simulink model "LIN_Edge"  (R2016b)
settings: Solver=FixedStepAuto  StartTime=0.0  StopTime=10  FixedStep=0.001  RelTol=1e-3
values from neighbouring files (symbols this model uses):
  A = [0, 1, 0; m*l_C*g*sqrt(2)/I_K, -C_psi/I_K, C_psi/I_K; 0, C_psi/I_R, -C_psi/I_R]    [ParameterInit.m]
  Ad = SSd.A    [ParameterInit.m]
  B = [0; -1/I_K; 1/I_R]    [ParameterInit.m]
  Bd = SSd.B    [ParameterInit.m]
  C = [0, 1, 0; 0, 0, 1]    [ParameterInit.m]
  Cd = SSd.C    [ParameterInit.m]
  Ta = 0.02    [ParameterInit.m]
undefined symbols (not defined in the file or in its folder): Kd, Ld, x_0, x_offset
libraries: simulink x1
settings Model: Creator=michael  LastModifiedBy=ich

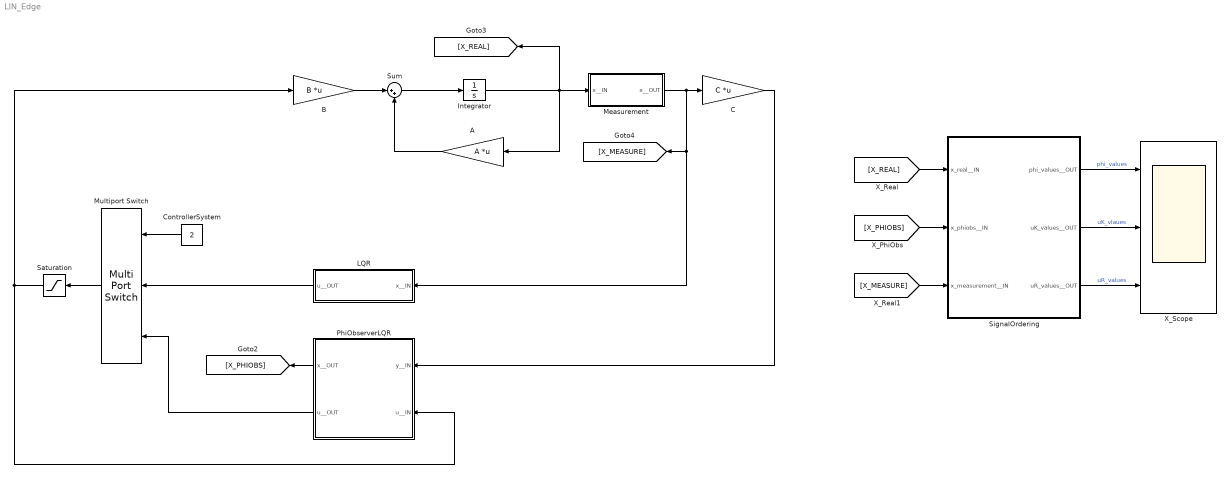
== system LIN_Edge ==
  A : Gain  Gain=A  Multiplication=Matrix(K*u) (u vector)
  B : Gain  Gain=B  Multiplication=Matrix(K*u) (u vector)
  C : Gain  Gain=C  Multiplication=Matrix(K*u) (u vector)
  ControllerSystem : Constant  Value=2
  Integrator : Integrator  InitialCondition=x_0
  LQR : Subsystem
  Measurement : Subsystem
  Multiport Switch : MultiPortSwitch  Inputs=2
  PhiObserverLQR : Subsystem
  Saturation : Saturate  UpperLimit=0.11  LowerLimit=-0.11
  SignalOrdering : Subsystem
  Sum : Sum  Inputs=|++
  X_Scope : Scope  NumInputPorts=3
  wires:
  B/1 -> Sum/1
  Sum/1 -> Integrator/1
  A/1 -> Sum/2
  Integrator/1 -> [X_REAL], Measurement/1(x__IN), A/1
  Measurement/1(x__OUT) -> C/1, LQR/1(x__IN), [X_MEASURE]
  Multiport Switch/1 -> Saturation/1
  LQR/1(u__OUT) -> Multiport Switch/2
  ControllerSystem/1 -> Multiport Switch/1
  Saturation/1 -> PhiObserverLQR/2(u__IN), B/1
  PhiObserverLQR/1(x__OUT) -> [X_PHIOBS]
  C/1 -> PhiObserverLQR/1(y__IN)
  [X_REAL] -> SignalOrdering/1(x_real__IN)
  [X_PHIOBS] -> SignalOrdering/2(x_phiobs__IN)
  [X_MEASURE] -> SignalOrdering/3(x_measurement__IN)
  SignalOrdering/1(phi_values__OUT) -> X_Scope/1  "phi_values"
  SignalOrdering/2(uK_values__OUT) -> X_Scope/2  "uK_vlaues"
  SignalOrdering/3(uR_values__OUT) -> X_Scope/3  "uR_values"
  PhiObserverLQR/2(u__OUT) -> Multiport Switch/3

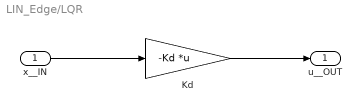
== system LIN_Edge/LQR ==
  x__IN : Inport  SampleTime=Ta
  Kd : Gain  Gain=-Kd  Multiplication=Matrix(K*u) (u vector)
  u__OUT : Outport
  wires:
  x__IN/1 -> Kd/1
  Kd/1 -> u__OUT/1

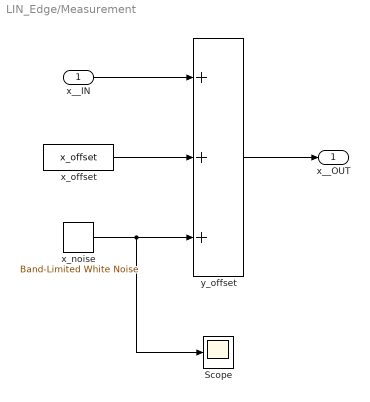
== system LIN_Edge/Measurement ==
  x__IN : Inport  SampleTime=Ta
  Scope : Scope
  x_noise : simulink/Sources/Band-Limited White Noise  Cov=y_noise  Ts=0.02  seed=[23341]
  x_offset : Constant  Value=x_offset
  y_offset : Sum  Inputs=+++
  x__OUT : Outport
  wires:
  x__IN/1 -> y_offset/1
  y_offset/1 -> x__OUT/1
  x_offset/1 -> y_offset/2
  x_noise/1 -> Scope/1, y_offset/3

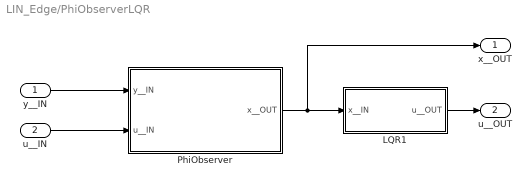
== system LIN_Edge/PhiObserverLQR ==
  y__IN : Inport
  u__IN : Inport  Port=2
  LQR1 : Subsystem
  PhiObserver : Subsystem
  x__OUT : Outport
  u__OUT : Outport  Port=2
  wires:
  LQR1/1(u__OUT) -> u__OUT/1
  PhiObserver/1(x__OUT) -> x__OUT/1, LQR1/1(x__IN)
  u__IN/1 -> PhiObserver/2(u__IN)
  y__IN/1 -> PhiObserver/1(y__IN)

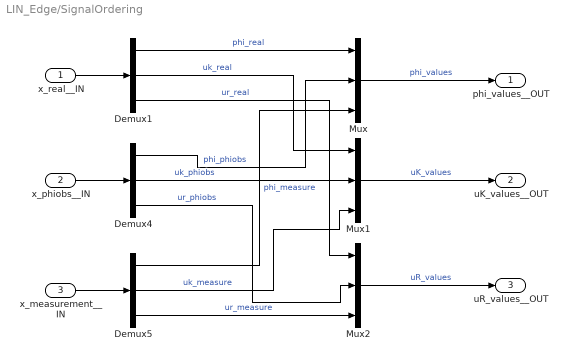
== system LIN_Edge/SignalOrdering ==
  x_real__IN : Inport
  x_phiobs__IN : Inport  Port=2
  x_measurement__IN : Inport  Port=3
  Demux1 : Demux  Outputs=3
  Demux4 : Demux  Outputs=3
  Demux5 : Demux  Outputs=3
  Mux : Mux  Inputs=3
  Mux1 : Mux  Inputs=3
  Mux2 : Mux  Inputs=3
  phi_values__OUT : Outport
  uK_values__OUT : Outport  Port=2
  uR_values__OUT : Outport  Port=3
  wires:
  Demux1/2 -> Mux1/1  "uk_real"
  Demux4/2 -> Mux1/2  "uk_phiobs"
  Demux4/3 -> Mux2/2  "ur_phiobs"
  x_real__IN/1 -> Demux1/1
  Mux/1 -> phi_values__OUT/1  "phi_values"
  Mux1/1 -> uK_values__OUT/1  "uK_values"
  Mux2/1 -> uR_values__OUT/1  "uR_values"
  Demux5/2 -> Mux1/3  "uk_measure"
  Demux1/1 -> Mux/1  "phi_real"
  x_measurement__IN/1 -> Demux5/1
  Demux4/1 -> Mux/2  "phi_phiobs"
  Demux1/3 -> Mux2/1  "ur_real"
  x_phiobs__IN/1 -> Demux4/1
  Demux5/1 -> Mux/3  "phi_measure"
  Demux5/3 -> Mux2/3  "ur_measure"

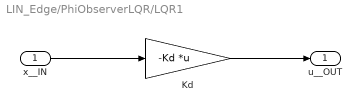
== system LIN_Edge/PhiObserverLQR/LQR1 ==
  x__IN : Inport  SampleTime=Ta
  Kd : Gain  Gain=-Kd  Multiplication=Matrix(K*u) (u vector)
  u__OUT : Outport
  wires:
  x__IN/1 -> Kd/1
  Kd/1 -> u__OUT/1

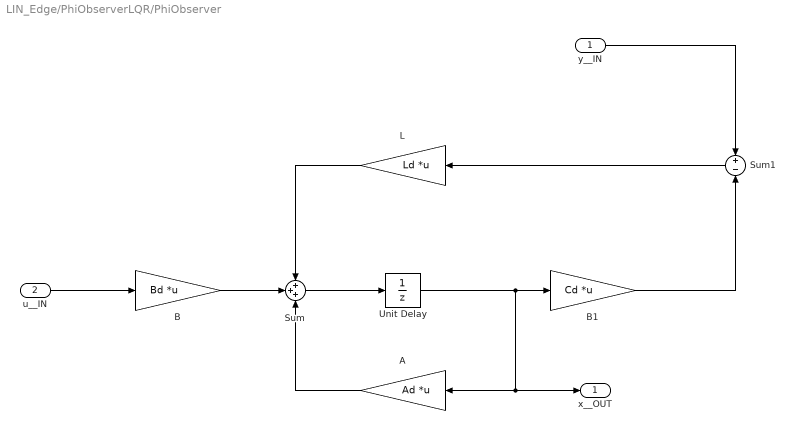
== system LIN_Edge/PhiObserverLQR/PhiObserver ==
  y__IN : Inport  SampleTime=Ta
  u__IN : Inport  Port=2  SampleTime=Ta
  A : Gain  Gain=Ad  Multiplication=Matrix(K*u) (u vector)
  B : Gain  Gain=Bd  Multiplication=Matrix(K*u) (u vector)
  B1 : Gain  Gain=Cd  Multiplication=Matrix(K*u) (u vector)
  L : Gain  Gain=Ld  Multiplication=Matrix(K*u) (u vector)
  Sum : Sum  Inputs=+++
  Sum1 : Sum  Inputs=+|-
  Unit Delay : UnitDelay  InitialCondition=[x_0+x_offset]  SampleTime=0.02
  x__OUT : Outport
  wires:
  y__IN/1 -> Sum1/1
  B1/1 -> Sum1/2
  Sum1/1 -> L/1
  Unit Delay/1 -> A/1, x__OUT/1, B1/1
  Sum/1 -> Unit Delay/1
  L/1 -> Sum/1
  A/1 -> Sum/3
  B/1 -> Sum/2
  u__IN/1 -> B/1
